simulink model "Control_Logic_b_chk2"  (R2019b)
settings: Solver=VariableStepAuto  StartTime=Start_time  StopTime=Stop_time  RelTol=1e-3
values from neighbouring files (symbols this model uses):
  Aset_N1 = 2    [Parameter_control.m]
  Aset_N10 = -10    [Parameter_control.m]
  Aset_N11 = 10    [Parameter_control.m]
  Aset_N12 = 20    [Parameter_control.m]
  Aset_N2 = 30    [Parameter_control.m]
  Aset_N3 = 3    [Parameter_control.m]
  Aset_N4 = 5    [Parameter_control.m]
  Aset_N5 = 1    [Parameter_control.m]
  Aset_N6 = 0    [Parameter_control.m]
  Aset_N7 = 0.01    [Parameter_control.m]
  Aset_N8 = 2    [Parameter_control.m]
  Aset_N9 = 0.1    [Parameter_control.m]
  Dset_N1 = 1    [Parameter_control.m]
  Dset_N2 = 1    [Parameter_control.m]
  Sample_time = 0.1    [main.m]    (also in test_tool_initialize.m)
undefined symbols (not defined in the file or in its folder): DiscIntNeverNeededParam
(part 3 of 3)

== matlab function Control_Logic_b_chk2/Velocity control/SUB/MATLAB Function ==
  data: u input; y output
% 減算器
function y = SUB(u)
    y = u(1) - u(2);

== matlab function Control_Logic_b_chk2/Velocity control/MUL1/MATLAB Function ==
  data: u input; y output
% 乗算器
function y = MUL(u)
    y = u(1) * u(2);

== matlab function Control_Logic_b_chk2/Velocity control/DIV1/MATLAB Function ==
  data: u input; y output; err output; set input
% 除算器
%       u(1), u(2) : 入力変数
%       set : FloatMax
%       y : 出力変数
function [y, err] = DIV(u, set)
    y = set;
    err = -1;
    if u(2) ~= 0
        y = u(1) / u(2);
        err = 1;
    end

== matlab function Control_Logic_b_chk2/Velocity control/SUB1/MATLAB Function ==
  data: u input; y output
% 減算器
function y = SUB(u)
    y = u(1) - u(2);

== matlab function Control_Logic_b_chk2/Velocity control/SUB2/MATLAB Function ==
  data: u input; y output
% 減算器
function y = SUB(u)
    y = u(1) - u(2);

== matlab function Control_Logic_b_chk2/Velocity control/HSS/MATLAB Function ==
  data: u input; y output
% 高値選択器
function y = HSS(u)
    y = u(1);
    if u(2) > y 
        y = u(2);
    end

== matlab function Control_Logic_b_chk2/Velocity control/LSS/MATLAB Function ==
  data: u input; y output
% 低値選択器
function y = LSS(u)
    y = u(1);
    if u(2) < y 
        y = u(2);
    end

== matlab function Control_Logic_b_chk2/Position control/BRLMT/MATLAB Function ==
  data: u input; y output; delta output; yold input; set input
% レートリミッタ
%   |(x-yold)/dt|＜変化レートならば、 y=x
%   |(x-yold)/dt|≧変化レートならば、 y=yold+変化レート
%       u：入力変数
%       yold：前回出力値
%       set(1)：変化レート
%       set(2)：計算刻み
%       y : 出力変数
function [y, delta] = BRLMT(u, yold, set)
    delta = (u - yold) / set(2);
    if (delta < set(1)) && (delta > -set(1))
        y = u;
    else
        if delta >= 0 
            y = yold + set(1) * set(2);
        else
            y = yold - set(1) * set(2);
        end
    end

== matlab function Control_Logic_b_chk2/Velocity control/BRLMT/MATLAB Function ==
  data: u input; y output; delta output; yold input; set input
% レートリミッタ
%   |(x-yold)/dt|＜変化レートならば、 y=x
%   |(x-yold)/dt|≧変化レートならば、 y=yold+変化レート
%       u：入力変数
%       yold：前回出力値
%       set(1)：変化レート
%       set(2)：計算刻み
%       y : 出力変数
function [y, delta] = BRLMT(u, yold, set)
    delta = (u - yold) / set(2);
    if (delta < set(1)) && (delta > -set(1))
        y = u;
    else
        if delta >= 0 
            y = yold + set(1) * set(2);
        else
            y = yold - set(1) * set(2);
        end
    end
